simulink model "Controller"  (R2015a)
settings: Solver=FixedStepDiscrete  StartTime=0.0  StopTime=10.0  FixedStep=delta_t  RelTol=1e-3
settings Model: Creator=Kerianne  LastModifiedBy=Kerianne
settings DataIOCC: SaveFormat=Structure
settings OptimizationCC: InlineParams=on  ExpressionDepthLimit=2147483647
settings DebuggingCC: UnderspecifiedInitializationDetection=Classic  MergeDetectMultiDrivingBlocksExec=none  SolverPrmCheckMsg=warning  StateNameClashWarn=warning

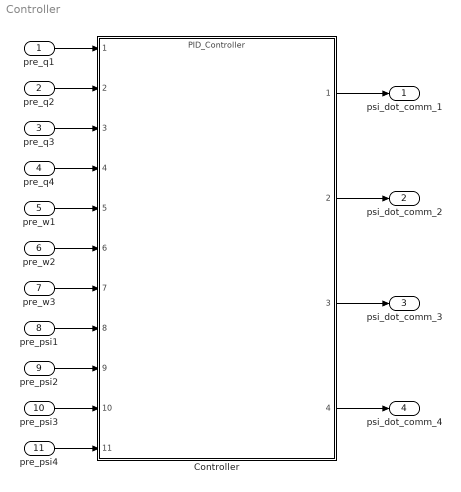
== system Controller ==
  pre_q1 : Inport
  pre_q2 : Inport  Port=2
  pre_q3 : Inport  Port=3
  pre_q4 : Inport  Port=4
  pre_w1 : Inport  Port=5
  pre_w2 : Inport  Port=6
  pre_w3 : Inport  Port=7
  pre_psi1 : Inport  Port=8
  pre_psi2 : Inport  Port=9
  pre_psi3 : Inport  Port=10
  pre_psi4 : Inport  Port=11
  Controller : ModelReference  ModelNameDialog=PID_Controller.slx  SimulationMode=Normal  ModelReferenceVersion=1.14  CopyOfModelName=PID_Controller.slx  DefaultDataLogging=on
  psi_dot_comm_1 : Outport
  psi_dot_comm_2 : Outport  Port=2
  psi_dot_comm_3 : Outport  Port=3
  psi_dot_comm_4 : Outport  Port=4
  wires:
  pre_q1/1 -> Controller/1
  pre_q2/1 -> Controller/2
  pre_q3/1 -> Controller/3
  pre_q4/1 -> Controller/4
  pre_w1/1 -> Controller/5
  pre_w2/1 -> Controller/6
  pre_w3/1 -> Controller/7
  pre_psi1/1 -> Controller/8
  pre_psi2/1 -> Controller/9
  pre_psi3/1 -> Controller/10
  Controller/3 -> psi_dot_comm_3/1
  Controller/2 -> psi_dot_comm_2/1
  Controller/1 -> psi_dot_comm_1/1
  Controller/4 -> psi_dot_comm_4/1
  pre_psi4/1 -> Controller/11
